simulink model "CubeQuat3"  (R2014a)
settings: Solver=ode45  StartTime=0.0  StopTime=5400  RelTol=1e-3
values from neighbouring files (symbols this model uses):
  adr = ADRblockGen(w,m,3)    [Control_mission_def.m]    (also in CubeSimSetUp.m; Example__simulaltion.m; Example_simulaltion.m; WBC_setup.m)
  distrej = 0    [Control_mission_def.m]    (also in CubeSimSetUp.m; Example__simulaltion.m; Example_simulaltion.m; WBC_setup.m = 1)
  I = diag(I_mom) + [0 I_prd(1) I_prd(2); I_prd(1) 0 I_prd(3); I_prd(2) I_prd(3) 0]    [CubeQuat_setup.m]    (also in CubeSatSfun.m = block.DialogPrm(2).Data; CubeSimSetUp.m = diag([Ixx;Iyy;Izz]); Satellite_Setup.m = diag([Ixx;Iyy;Izz]); Satellite_Setup_Sun_Pointing.m = diag([Ixx;Iyy;Izz]))
  k = 1e-6    (= 1e-06)    [Control_mission_def.m]    (also in CubeSimSetUp.m; Example__simulaltion.m = 1e-09; Example_simulaltion.m = 5e-08; WBC_setup.m = 5e-09)
  kd = 6e-4    (= 0.0006)    [Control_mission_def.m]    (also in CubeQuat_setup.m = 2*sqrt(I(1,1))*sqrt(kp); CubeSimSetUp.m; Example__simulaltion.m; Example_simulaltion.m)
  kp = 5e-9    (= 5e-09)    [Control_mission_def.m]    (also in CubeQuat_setup.m = 40; CubeSimSetUp.m; Example__simulaltion.m; Example_simulaltion.m)
  omega_0 = [30;30;30]*(1/sqrt(3))*(pi/180)    [CubeQuat_setup.m]
  omega_orbit = [0;-7.67/(401.1+6371);0]    [CubeQuat_setup.m]    (also in CubeSatSfun.m = block.DialogPrm(3).Data; CubeSimSetUp.m; Satellite_Setup.m; Satellite_Setup_Sun_Pointing.m)
  q_ref = q_3_ref    [Control_mission_def.m]    (also in CubeSimSetUp.m = angle2quat(0,0,0,'XYZ'); Example__simulaltion.m; Example_simulaltion.m; WS_20_09_2017.mat = [0.707106781187 0.707106781187 0 0])
  x_0 = [0,0,0,1,0,0,0]    [CubeQuat_setup.m]    (also in CubeSimSetUp.m = [wb_bi_init;qb_o_init;qb_i_init;qo_i_init;long_init;lat_init; Example__simulaltion.m = transpose([wb_bi_init,qb_i_init]); Example_simulaltion.m = transpose([wb_bi_init,qb_i_init]); Satellite_Setup.m = transpose([wb_bi_init,qb_i_init]))
libraries: cstblocks x12, aerolibtransform2 x6
settings Model: Creator=Daire  LastModifiedBy=Daire

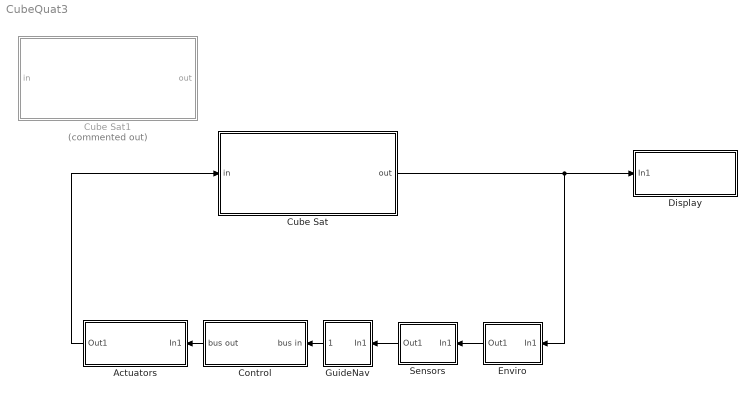
== system CubeQuat3 ==
  Actuators : Subsystem
  Control : Subsystem  Variant=on
  Cube Sat : Subsystem
  Cube Sat1 : Subsystem  Commented=on
  Display : Subsystem
  Enviro : Subsystem
  GuideNav : Subsystem
  Sensors : Subsystem
  wires:
  Cube Sat/1(out) -> Enviro/1(In1), Display/1(In1)
  Sensors/1(Out1) -> GuideNav/1(In1)
  Control/1(bus out) -> Actuators/1(In1)
  Actuators/1(Out1) -> Cube Sat/1(in)
  GuideNav/1(Out1) -> Control/1(bus in)
  Enviro/1(Out1) -> Sensors/1(In1)

== system CubeQuat3/Actuators ==
  In1 : Inport
  Out1 : Outport
  wires:
  In1/1 -> Out1/1

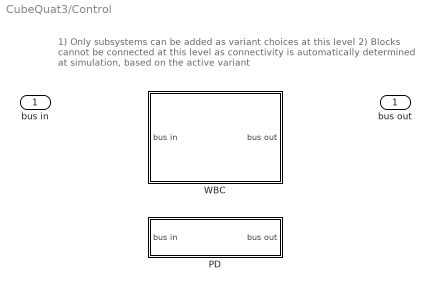
== system CubeQuat3/Control ==
  note: 1) Only subsystems can be added as variant choices at this level
      | 2) Blocks cannot be connected at this level as connectivity is
      | automatically determined at simulation, based on the active variant
  bus in : Inport
  PD : Subsystem  VariantControl=CtrlType==2
  WBC : Subsystem  VariantControl=CtrlType==1
  bus out : Outport

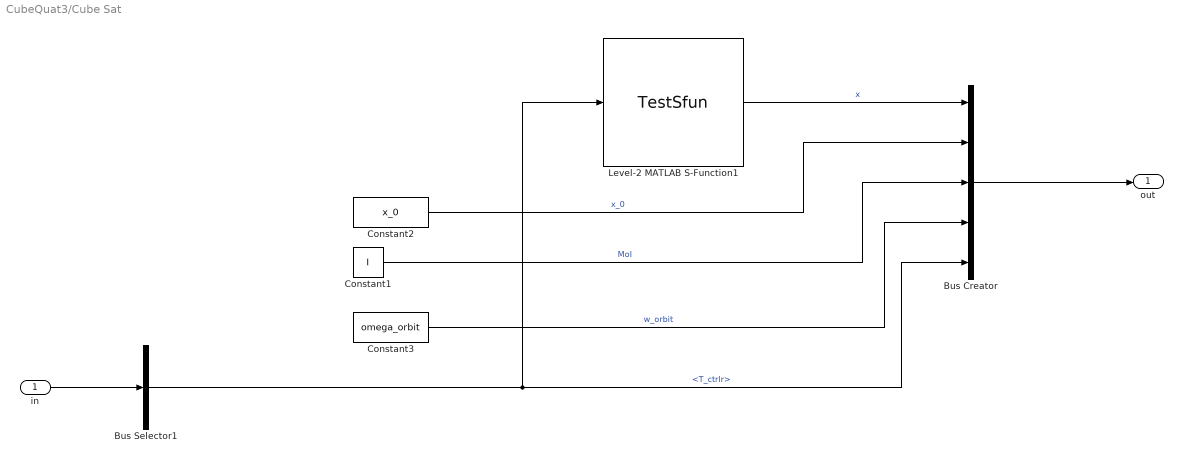
== system CubeQuat3/Cube Sat ==
  in : Inport
  Bus Creator : BusCreator  Inputs=5
  Bus Selector1 : BusSelector  OutputSignals=T_ctrlr
  Constant1 : Constant  Value=I
  Constant2 : Constant  Value=x_0
  Constant3 : Constant  Value=omega_orbit
  Level-2 MATLAB S-Function1 : M-S-Function  FunctionName=TestSfun  Parameters=x_0,I,omega_0  mask{Parameter2=x_0, Parameter3=I, Parameter4=omega_orbit}
      mask prompts: Parameter2 "x_0"; Parameter3 "I"; Parameter4 "omega_orbit"
      mask Display:
      | disp('Cube Sat Model')
      | port_label('input',1,'T')
      | port_label('output',1,'x')
  out : Outport
  wires:
  Constant1/1 -> Bus Creator/3  "MoI"
  Constant3/1 -> Bus Creator/4  "w_orbit"
  Bus Creator/1 -> out/1
  in/1 -> Bus Selector1/1
  Bus Selector1/1 -> Level-2 MATLAB S-Function1/1, Bus Creator/5  "<T_ctrlr>"
  Level-2 MATLAB S-Function1/1 -> Bus Creator/1  "x"
  Constant2/1 -> Bus Creator/2  "x_0"

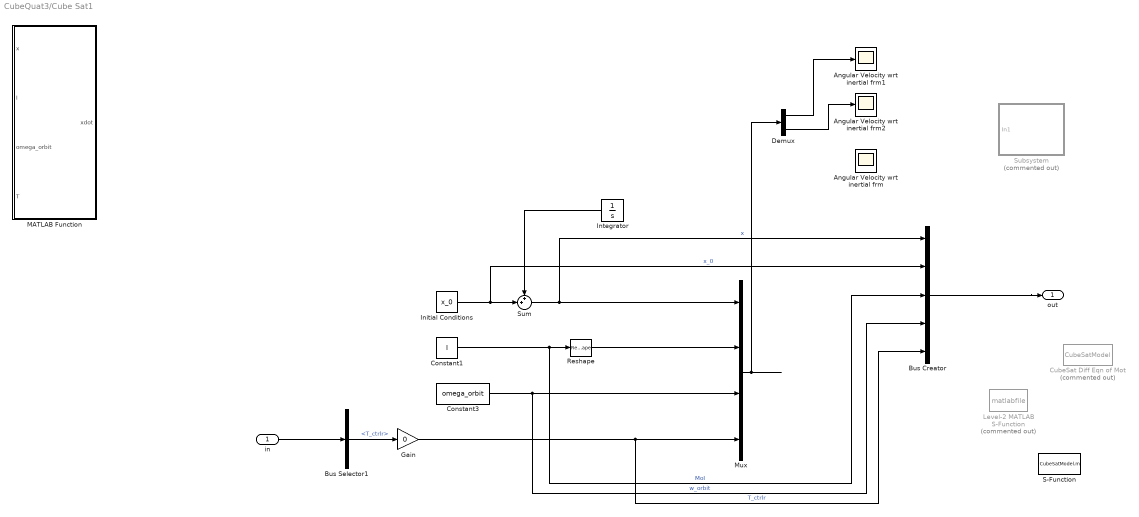
== system CubeQuat3/Cube Sat1 ==
  in : Inport
  Angular Velocity wrt inertial frm : Scope
      settings: ShowLegends=on  SaveName=ScopeData13
  Angular Velocity wrt inertial frm1 : Scope
      settings: ShowLegends=on  SaveName=ScopeData14
  Angular Velocity wrt inertial frm2 : Scope
      settings: ShowLegends=on  SaveName=ScopeData15
  Bus Creator : BusCreator  Inputs=5
  Bus Selector1 : BusSelector  OutputSignals=T_ctrlr
  Constant1 : Constant  Value=I
  Constant3 : Constant  Value=omega_orbit
  CubeSat Diff Eqn of Mot : MATLABFcn  Commented=on  MATLABFcn=CubeSatModel
  Demux : Demux  Outputs=2
  Gain : Gain  Gain=0
  Initial Conditions : Constant  Value=x_0
  Integrator : Integrator
  Level-2 MATLAB S-Function : M-S-Function  Commented=on
  MATLAB Function : MATLAB Function  TreatAsAtomicUnit=on
  Mux : Mux
  Reshape : Reshape
  S-Function : S-Function  FunctionName=CubeSatModel.m  EnableBusSupport=off
  Subsystem : Subsystem  Commented=on
  Sum : Sum  Inputs=++|
  out : Outport
  wires:
  Demux/2 -> Angular Velocity wrt inertial frm2/1
  Demux/1 -> Angular Velocity wrt inertial frm1/1
  Reshape/1 -> Mux/2
  Mux/1 -> Demux/1
  Bus Selector1/1 -> Gain/1  "<T_ctrlr>"
  in/1 -> Bus Selector1/1
  Gain/1 -> Bus Creator/5, Mux/4  "T_ctrlr"
  Bus Creator/1 -> out/1
  Constant3/1 -> Mux/3, Bus Creator/4  "w_orbit"
  Constant1/1 -> Reshape/1, Bus Creator/3  "MoI"
  Initial Conditions/1 -> Sum/2, Bus Creator/2  "x_0"
  ? -> Integrator/1, Angular Velocity wrt inertial frm/1  "x_dot"
  Sum/1 -> Bus Creator/1, Mux/1  "x"
  Integrator/1 -> Sum/1

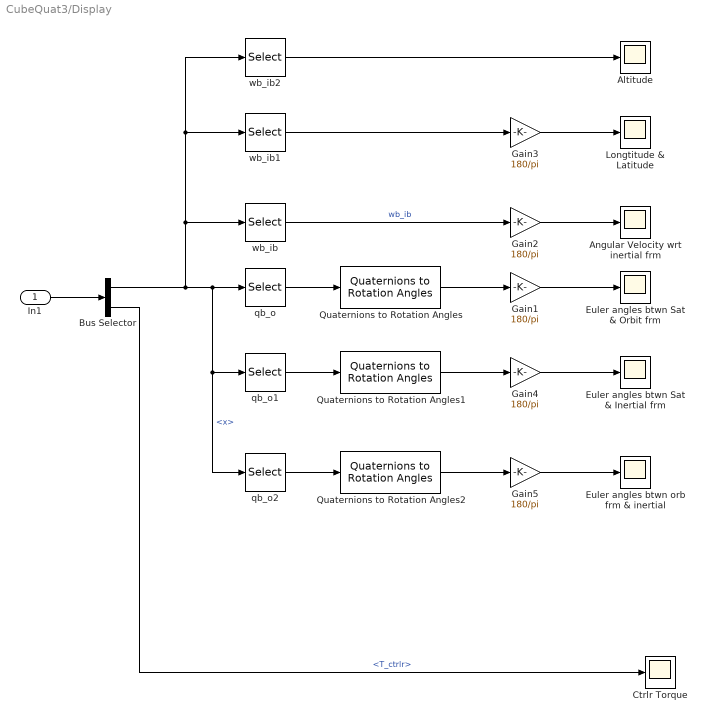
== system CubeQuat3/Display ==
  In1 : Inport
  Altitude : Scope
      settings: SaveName=ScopeData5
  Angular Velocity wrt inertial frm : Scope
  Bus Selector : BusSelector  OutputSignals=x,T_ctrlr
  Ctrlr Torque : Scope
      settings: SaveName=ScopeData2
  Euler angles btwn Sat & Inertial frm : Scope
      settings: SaveName=ScopeData4
  Euler angles btwn Sat & Orbit frm : Scope
  Euler angles btwn orb frm & inertial : Scope
      settings: SaveName=ScopeData6
  Gain{1..5} (5 alike) : Gain  Gain=180/pi
  Longtitude & Latitude : Scope
      settings: SaveName=ScopeData3
  Quaternions to Rotation Angles : aerolibtransform2/Quaternions to Rotation Angles  rotationOrder=ZYX
  Quaternions to Rotation Angles1 : aerolibtransform2/Quaternions to Rotation Angles  rotationOrder=ZYX
  Quaternions to Rotation Angles2 : aerolibtransform2/Quaternions to Rotation Angles  rotationOrder=ZYX
  qb_o : Selector  InputPortWidth=18  Indices=[4,5,6,7]
  qb_o1 : Selector  InputPortWidth=18  Indices=[8,9,10,11]
  qb_o2 : Selector  InputPortWidth=18  Indices=[8,9,10,11]
  wb_ib : Selector  InputPortWidth=18  Indices=[1,2,3]
  wb_ib1 : Selector  InputPortWidth=18  Indices=[16,17]
  wb_ib2 : Selector  InputPortWidth=18  Indices=[18]
  wires:
  In1/1 -> Bus Selector/1
  Bus Selector/2 -> Ctrlr Torque/1  "<T_ctrlr>"
  qb_o/1 -> Quaternions to Rotation Angles/1
  wb_ib/1 -> Gain2/1  "wb_ib"
  Quaternions to Rotation Angles/1 -> Gain1/1
  Gain2/1 -> Angular Velocity wrt inertial frm/1
  Gain1/1 -> Euler angles btwn Sat & Orbit frm/1
  wb_ib1/1 -> Gain3/1
  Gain3/1 -> Longtitude & Latitude/1
  qb_o1/1 -> Quaternions to Rotation Angles1/1
  Quaternions to Rotation Angles1/1 -> Gain4/1
  Gain4/1 -> Euler angles btwn Sat & Inertial frm/1
  wb_ib2/1 -> Altitude/1
  Bus Selector/1 -> wb_ib2/1, wb_ib1/1, wb_ib/1, qb_o2/1, qb_o1/1, qb_o/1  "<x>"
  qb_o2/1 -> Quaternions to Rotation Angles2/1
  Quaternions to Rotation Angles2/1 -> Gain5/1
  Gain5/1 -> Euler angles btwn orb frm & inertial/1

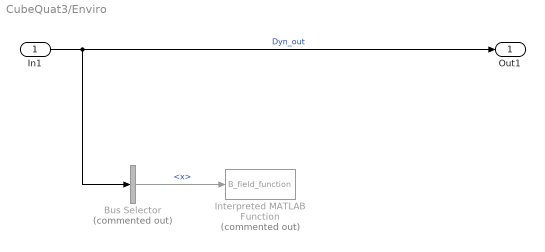
== system CubeQuat3/Enviro ==
  In1 : Inport
  Bus Selector : BusSelector  Commented=on  OutputSignals=x
  Interpreted MATLAB Function : MATLABFcn  Commented=on  MATLABFcn=B_field_function
  Out1 : Outport
  wires:
  In1/1 -> Out1/1, Bus Selector/1  "Dyn_out"
  Bus Selector/1 -> Interpreted MATLAB Function/1  "<x>"

== system CubeQuat3/GuideNav ==
  In1 : Inport
  Bus Creator : BusCreator  Inputs=2
  Constant : Constant  Value=q_ref
  Out1 : Outport
  wires:
  In1/1 -> Bus Creator/1  "Sensor_out"
  Bus Creator/1 -> Out1/1
  Constant/1 -> Bus Creator/2  "q_ref"

== system CubeQuat3/Sensors ==
  In1 : Inport
  Out1 : Outport
  wires:
  In1/1 -> Out1/1

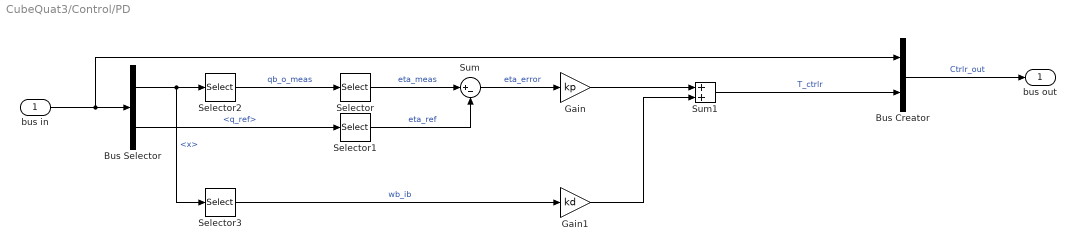
== system CubeQuat3/Control/PD ==
  bus in : Inport
  Bus Creator : BusCreator  Inputs=2
  Bus Selector : BusSelector  OutputSignals=Sensor_out.x,q_ref
  Gain : Gain  Gain=kp
  Gain1 : Gain  Gain=kd
  Selector : Selector  InputPortWidth=4  Indices=[2 3 4]
  Selector1 : Selector  InputPortWidth=4  Indices=[2 3 4]
  Selector2 : Selector  InputPortWidth=18  Indices=[4;5;6;7]
  Selector3 : Selector  InputPortWidth=18  Indices=[1,2,3]
  Sum : Sum  Inputs=|+-
  Sum1 : Sum
  bus out : Outport
  wires:
  bus in/1 -> Bus Creator/1, Bus Selector/1
  Bus Selector/2 -> Selector1/1  "<q_ref>"
  Selector2/1 -> Selector/1  "qb_o_meas"
  Bus Selector/1 -> Selector3/1, Selector2/1  "<x>"
  Selector/1 -> Sum/1  "eta_meas"
  Selector1/1 -> Sum/2  "eta_ref"
  Sum/1 -> Gain/1  "eta_error"
  Gain/1 -> Sum1/1
  Sum1/1 -> Bus Creator/2  "T_ctrlr"
  Bus Creator/1 -> bus out/1  "Ctrlr_out"
  Selector3/1 -> Gain1/1  "wb_ib"
  Gain1/1 -> Sum1/2

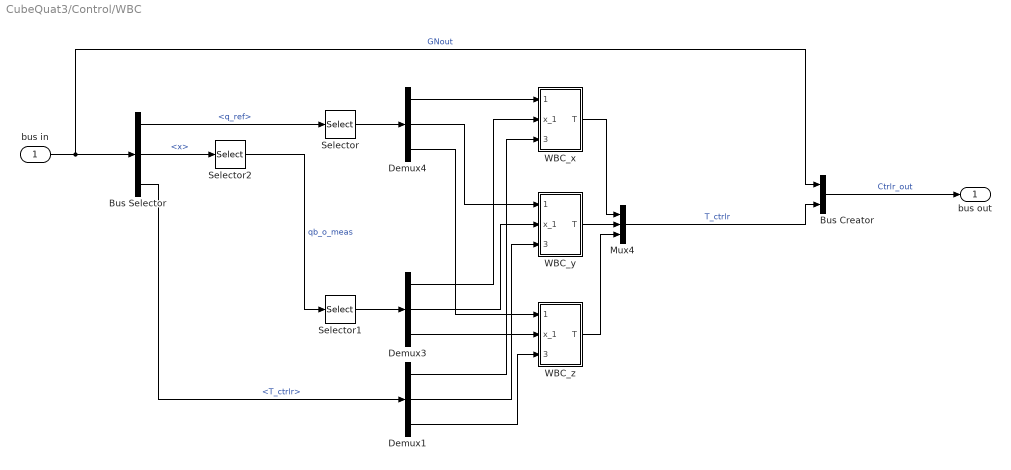
== system CubeQuat3/Control/WBC ==
  bus in : Inport
  Bus Creator : BusCreator  Inputs=2
  Bus Selector : BusSelector  OutputSignals=q_ref,Sensor_out.x,Sensor_out.T_ctrlr
  Demux1 : Demux  Outputs=3
  Demux3 : Demux  Outputs=3
  Demux4 : Demux  Outputs=3
  Mux4 : Mux  Inputs=3
  Selector : Selector  InputPortWidth=4  Indices=[2 3 4]
  Selector1 : Selector  InputPortWidth=4  Indices=[2 3 4]
  Selector2 : Selector  InputPortWidth=18  Indices=[4,5,6,7]
  WBC_x : Subsystem
  WBC_y : Subsystem
  WBC_z : Subsystem
  bus out : Outport
  wires:
  Demux3/3 -> WBC_z/2(x_1)
  Bus Selector/2 -> Selector2/1  "<x>"
  WBC_y/1(T) -> Mux4/2
  Mux4/1 -> Bus Creator/2  "T_ctrlr"
  WBC_z/1(T) -> Mux4/3
  WBC_x/1(T) -> Mux4/1
  Demux3/2 -> WBC_y/2(x_1)
  Demux3/1 -> WBC_x/2(x_1)
  Bus Selector/3 -> Demux1/1  "<T_ctrlr>"
  Demux1/1 -> WBC_x/3(T_meas)
  Demux1/2 -> WBC_y/3(T_meas)
  Demux1/3 -> WBC_z/3(T_meas)
  Demux4/1 -> WBC_x/1(x_0_ref)
  Demux4/3 -> WBC_z/1(x_0_ref)
  Demux4/2 -> WBC_y/1(x_0_ref)
  Selector/1 -> Demux4/1
  Selector1/1 -> Demux3/1
  bus in/1 -> Bus Creator/1, Bus Selector/1  "GNout"
  Bus Selector/1 -> Selector/1  "<q_ref>"
  Bus Creator/1 -> bus out/1  "Ctrlr_out"
  Selector2/1 -> Selector1/1  "qb_o_meas"

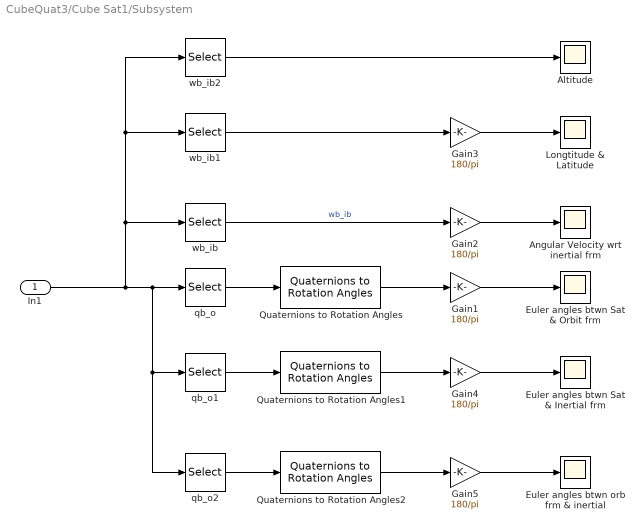
== system CubeQuat3/Cube Sat1/Subsystem ==
  In1 : Inport
  Altitude : Scope
      settings: SaveName=ScopeData7
  Angular Velocity wrt inertial frm : Scope
      settings: SaveName=ScopeData8
  Euler angles btwn Sat & Inertial frm : Scope
      settings: SaveName=ScopeData9
  Euler angles btwn Sat & Orbit frm : Scope
      settings: SaveName=ScopeData10
  Euler angles btwn orb frm & inertial : Scope
      settings: SaveName=ScopeData11
  Gain{1..5} (5 alike) : Gain  Gain=180/pi
  Longtitude & Latitude : Scope
      settings: SaveName=ScopeData12
  Quaternions to Rotation Angles : aerolibtransform2/Quaternions to Rotation Angles  rotationOrder=ZYX
  Quaternions to Rotation Angles1 : aerolibtransform2/Quaternions to Rotation Angles  rotationOrder=ZYX
  Quaternions to Rotation Angles2 : aerolibtransform2/Quaternions to Rotation Angles  rotationOrder=ZYX
  qb_o : Selector  InputPortWidth=18  Indices=[4,5,6,7]
  qb_o1 : Selector  InputPortWidth=18  Indices=[8,9,10,11]
  qb_o2 : Selector  InputPortWidth=18  Indices=[8,9,10,11]
  wb_ib : Selector  InputPortWidth=18  Indices=[1,2,3]
  wb_ib1 : Selector  InputPortWidth=18  Indices=[16,17]
  wb_ib2 : Selector  InputPortWidth=18  Indices=[18]
  wires:
  Gain5/1 -> Euler angles btwn orb frm & inertial/1
  Quaternions to Rotation Angles2/1 -> Gain5/1
  wb_ib2/1 -> Altitude/1
  qb_o2/1 -> Quaternions to Rotation Angles2/1
  In1/1 -> qb_o/1, qb_o1/1, qb_o2/1, wb_ib/1, wb_ib1/1, wb_ib2/1
  Gain4/1 -> Euler angles btwn Sat & Inertial frm/1
  wb_ib1/1 -> Gain3/1
  Gain1/1 -> Euler angles btwn Sat & Orbit frm/1
  Quaternions to Rotation Angles1/1 -> Gain4/1
  qb_o1/1 -> Quaternions to Rotation Angles1/1
  Gain3/1 -> Longtitude & Latitude/1
  Gain2/1 -> Angular Velocity wrt inertial frm/1
  Quaternions to Rotation Angles/1 -> Gain1/1
  wb_ib/1 -> Gain2/1  "wb_ib"
  qb_o/1 -> Quaternions to Rotation Angles/1

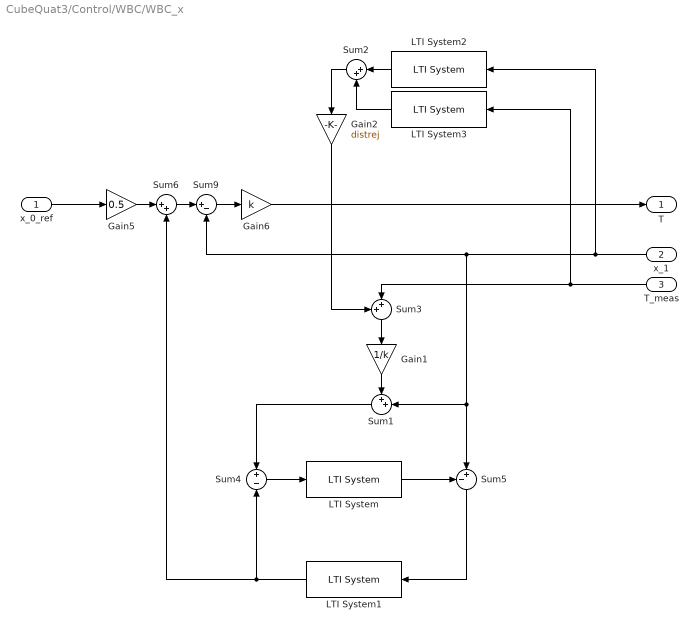
== system CubeQuat3/Control/WBC/WBC_x ==
  x_0_ref : Inport
  x_1 : Inport  Port=2
  T_meas : Inport  Port=3
  Gain1 : Gain  Gain=1/k
  Gain2 : Gain  Gain=distrej
  Gain5 : Gain  Gain=0.5
  Gain6 : Gain  Gain=k
  LTI System : cstblocks/LTI System  sys=G  IC=[]
  LTI System1 : cstblocks/LTI System  sys=G  IC=[]
  LTI System2 : cstblocks/LTI System  sys=adr(1)  IC=[]
  LTI System3 : cstblocks/LTI System  sys=adr(2)  IC=[]
  Sum1 : Sum  Inputs=++|
  Sum2 : Sum  Inputs=|++
  Sum3 : Sum  Inputs=++|
  Sum4 : Sum  Inputs=+|-
  Sum5 : Sum  Inputs=-+|
  Sum6 : Sum  Inputs=|++
  Sum9 : Sum  Inputs=|+-
  T : Outport
  wires:
  Sum1/1 -> Sum4/1
  Gain1/1 -> Sum1/1
  x_1/1 -> Sum1/2, Sum5/2, Sum9/2, LTI System2/1
  Sum5/1 -> LTI System1/1
  LTI System/1 -> Sum5/1
  Sum4/1 -> LTI System/1
  LTI System1/1 -> Sum4/2, Sum6/2
  Gain5/1 -> Sum6/1
  Gain6/1 -> T/1
  Sum9/1 -> Gain6/1
  Sum6/1 -> Sum9/1
  LTI System2/1 -> Sum2/1
  LTI System3/1 -> Sum2/2
  Sum2/1 -> Gain2/1
  Sum3/1 -> Gain1/1
  Gain2/1 -> Sum3/1
  x_0_ref/1 -> Gain5/1
  T_meas/1 -> Sum3/2, LTI System3/1

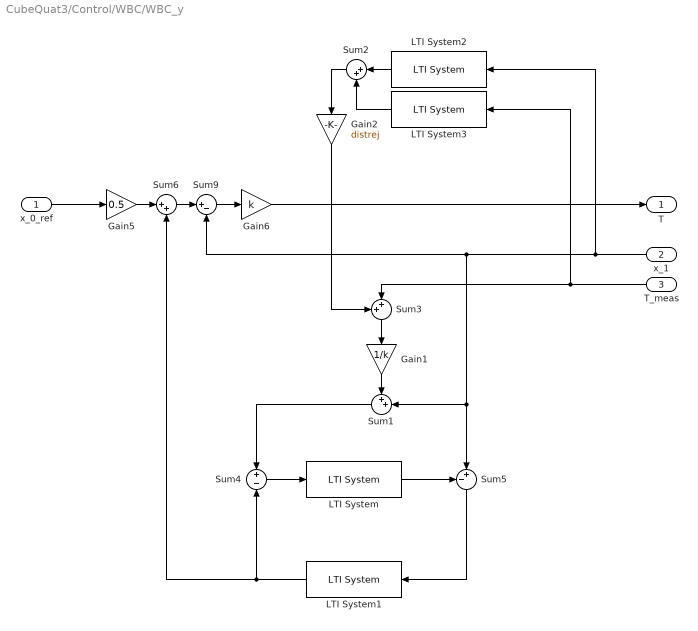
== system CubeQuat3/Control/WBC/WBC_y ==
  x_0_ref : Inport
  x_1 : Inport  Port=2
  T_meas : Inport  Port=3
  Gain1 : Gain  Gain=1/k
  Gain2 : Gain  Gain=distrej
  Gain5 : Gain  Gain=0.5
  Gain6 : Gain  Gain=k
  LTI System : cstblocks/LTI System  sys=G  IC=[]
  LTI System1 : cstblocks/LTI System  sys=G  IC=[]
  LTI System2 : cstblocks/LTI System  sys=adr(1)  IC=[]
  LTI System3 : cstblocks/LTI System  sys=adr(2)  IC=[]
  Sum1 : Sum  Inputs=++|
  Sum2 : Sum  Inputs=|++
  Sum3 : Sum  Inputs=++|
  Sum4 : Sum  Inputs=+|-
  Sum5 : Sum  Inputs=-+|
  Sum6 : Sum  Inputs=|++
  Sum9 : Sum  Inputs=|+-
  T : Outport
  wires:
  T_meas/1 -> LTI System3/1, Sum3/2
  x_0_ref/1 -> Gain5/1
  Gain2/1 -> Sum3/1
  Sum3/1 -> Gain1/1
  Sum2/1 -> Gain2/1
  LTI System3/1 -> Sum2/2
  LTI System2/1 -> Sum2/1
  Sum6/1 -> Sum9/1
  Sum9/1 -> Gain6/1
  Gain6/1 -> T/1
  Gain5/1 -> Sum6/1
  LTI System1/1 -> Sum6/2, Sum4/2
  Sum4/1 -> LTI System/1
  LTI System/1 -> Sum5/1
  Sum5/1 -> LTI System1/1
  x_1/1 -> LTI System2/1, Sum9/2, Sum5/2, Sum1/2
  Gain1/1 -> Sum1/1
  Sum1/1 -> Sum4/1

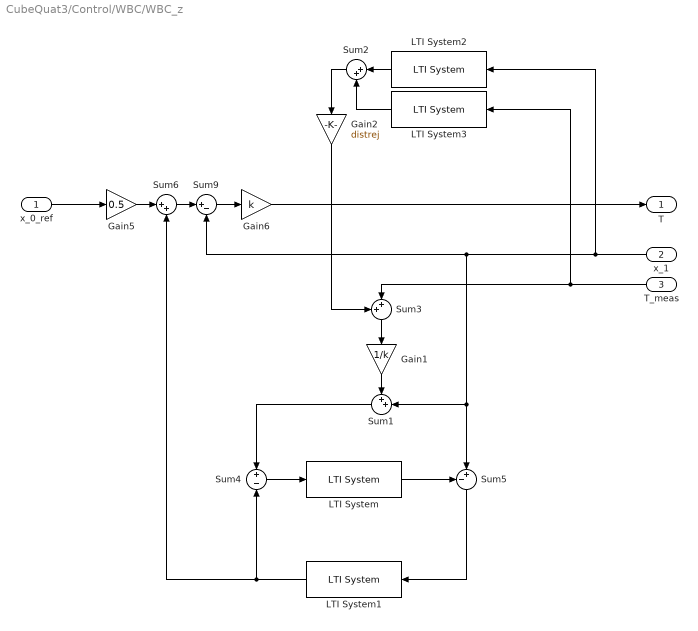
== system CubeQuat3/Control/WBC/WBC_z ==
  x_0_ref : Inport
  x_1 : Inport  Port=2
  T_meas : Inport  Port=3
  Gain1 : Gain  Gain=1/k
  Gain2 : Gain  Gain=distrej
  Gain5 : Gain  Gain=0.5
  Gain6 : Gain  Gain=k
  LTI System : cstblocks/LTI System  sys=G  IC=[]
  LTI System1 : cstblocks/LTI System  sys=G  IC=[]
  LTI System2 : cstblocks/LTI System  sys=adr(1)  IC=[]
  LTI System3 : cstblocks/LTI System  sys=adr(2)  IC=[]
  Sum1 : Sum  Inputs=++|
  Sum2 : Sum  Inputs=|++
  Sum3 : Sum  Inputs=++|
  Sum4 : Sum  Inputs=+|-
  Sum5 : Sum  Inputs=-+|
  Sum6 : Sum  Inputs=|++
  Sum9 : Sum  Inputs=|+-
  T : Outport
  wires:
  Sum1/1 -> Sum4/1
  Gain1/1 -> Sum1/1
  x_1/1 -> Sum1/2, Sum5/2, Sum9/2, LTI System2/1
  Sum5/1 -> LTI System1/1
  LTI System/1 -> Sum5/1
  Sum4/1 -> LTI System/1
  LTI System1/1 -> Sum4/2, Sum6/2
  Gain5/1 -> Sum6/1
  Gain6/1 -> T/1
  Sum9/1 -> Gain6/1
  Sum6/1 -> Sum9/1
  LTI System2/1 -> Sum2/1
  LTI System3/1 -> Sum2/2
  Sum2/1 -> Gain2/1
  Sum3/1 -> Gain1/1
  Gain2/1 -> Sum3/1
  x_0_ref/1 -> Gain5/1
  T_meas/1 -> Sum3/2, LTI System3/1

== matlab function CubeQuat3/Cube Sat1/MATLAB Function ==
  data: x input; xdot output; I input; omega_orbit input; T input
function xdot   = CubeQuat3(x,I,omega_orbit,T)
%Model of orbiting cube sat dynamics
%   A model a cube sat orbing the earth. The output, xdot, is the time
%   derivative of the state vector x. x=[omega;qb_i;qb_o;qo_i]. where omega is the
%   angular velocity of the body fixed frame relative to the inertial frame
%   at the centre of the earth. qb_i is a quaternion which represents the
%   rotation between the body fixed frame and the orbital plane. qb_o is
%   the quaternion representing the rotation between body and inertial
%   frame. qo_i is that relating orbital and inertial frames.

%% state info

% current state vector
omegab_ib=x(1:3);%angular vel of bod frame wrt inert frame
% quaternion rep rotation between body frame and orbit frame
q_o=x(4:7);
n_o=q_o(1);
eta_o=q_o(2:4);
% quaternion re rotation between body frame and inertial frame
q_i=x(8:11);
n_i=q_i(1);
eta_i=q_i(2:4);

%quat rep rotation between orbital frame and inertial frame
qoi=x(12:15);
n_oi=qoi(1);
eta_oi=qoi(2:4);

long=x(16);% From West to East (+-180) East is pos
lat=x(17);% From North to South (+-90deg) North is pos
Alt=x(18);



%% rotaton between frames

% between body and orbit frame
S_o=SkewSym(eta_o);
Ro_b=eye(3)+(2*n_o*S_o)+(2*(S_o^2));%from body to orbit frame
Rb_o=transpose(Ro_b);%from orbit to body frame
c_3=Rb_o(:,3);%needed for gravity gradient


% between body and inertial frames
S_i=SkewSym(eta_i);
Ri_b=eye(3)+(2*n_i*S_i)+(2*(S_i^2));%from body to inertial frame
Rb_i=transpose(Ri_b);

% between orbital and inertial
Ro_i=Ro_b*Rb_i;
Ri_o=transpose(Ro_i);
%er_i=Ri_o*[0.1;0.2;0.3];

% define the angular velocity of the body frame wrt orbital frame.
omegab_ob=omegab_ib-(Rb_o*omega_orbit);
S_oi=SkewSym(eta_oi);



%% Differential Equations of Motion

%derivative of omega of body frame wrt inertial frame
omega_ib_dot=I\(-cross(omegab_ib,I*omegab_ib)+T);%+T_ext);
%q meas wrt orbit frame
n_o_dot=-0.5*transpose(eta_o)*omegab_ob;
eta_o_dot=0.5*((n_o*eye(3))+S_o)*omegab_ob;
%q meas wrt inertial frame
n_i_dot=-0.5*transpose(eta_i)*omegab_ib;
eta_i_dot=0.5*((n_i*eye(3))+S_i)*omegab_ib;
%q representing rotation between orbital n inertail frame
noidot=-0.5*transpose(eta_oi)*omega_orbit;
etaoidot=0.5*((n_oi*eye(3))+S_oi)*omega_orbit;

long_dot=omega_orbit(2);
lat_dot=sqrt((omega_orbit(1)^2)+(omega_orbit(3)^2));
Alt_dot=0;%const altitude

xdot=[omega_ib_dot;n_o_dot;eta_o_dot;n_i_dot;eta_i_dot;noidot;etaoidot;long_dot;lat_dot;Alt_dot];

end
